simulink model "Simulator_Unitree_A1"  (R2022b)
settings: Solver=VariableStepAuto  StartTime=0.0  StopTime=70  RelTol=1e-3
undefined symbols (not defined in the file or in its folder): g, h, Kwalk, stepHeight, TsCtrl, tWalk, X, Y, Z
libraries: sm_lib x175, nesl_utility x69, simulink x2, slpidlib x2
(part 1 of 4)
settings Model: Creator=MUN  LastModifiedBy=MUN
settings ModelReferenceCC: EnableRefExpFcnMdlSchedulingChecks=on

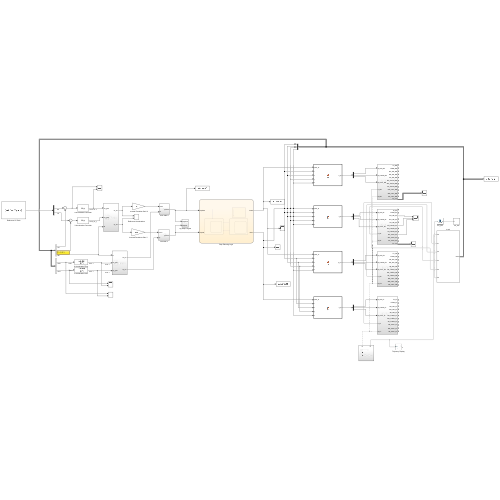
[thumbnail: Simulink's stored preview of the top-level diagram]
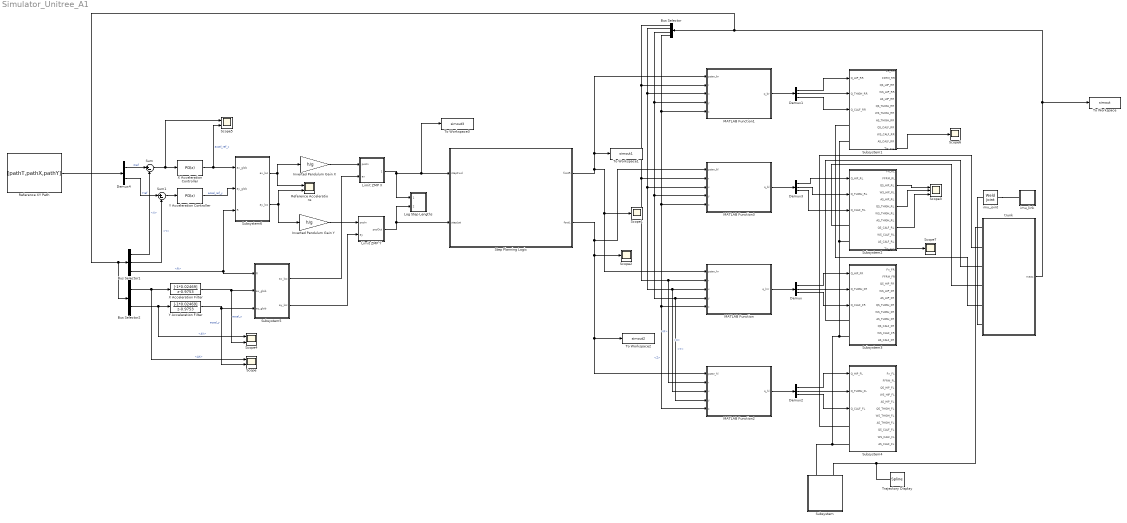
== system Simulator_Unitree_A1 ==
  Bus Selector : BusSelector  OutputSignals=R,X,Y,Z
  Bus Selector1 : BusSelector  OutputSignals=X,Y,R
  Bus Selector2 : BusSelector  OutputSignals=AX,AY
  Demux{,1..3} (4 alike) : Demux  Outputs=3
  Demux4 : Demux  Outputs=2
  Inverted Pendulum Gain X : Gain  Gain=h/g
  Inverted Pendulum Gain Y : Gain  Gain=h/g
  Limit ZMP X : Subsystem
  Limit ZMP Y : Subsystem
  Log Step Lengths : Subsystem
  MATLAB Function : MATLAB Function  TreatAsAtomicUnit=on
  MATLAB Function1 : MATLAB Function  TreatAsAtomicUnit=on
  MATLAB Function2 : MATLAB Function  TreatAsAtomicUnit=on
  MATLAB Function3 : MATLAB Function  TreatAsAtomicUnit=on
  Reference Accelerations : Scope  NumInputPorts=2
  Reference XY Path : FromWorkspace  VariableName=[pathT,pathX,pathY]  SampleTime=TsCtrl  OutputAfterFinalValue=Holding final value
  Scope : Scope  NumInputPorts=2
  Scope{1..2,6..7} (4 alike) : Scope
  Scope3 : Scope  NumInputPorts=3
  Scope4 : Scope  NumInputPorts=2
  Scope5 : Scope  NumInputPorts=2
  Step Planning Logic : Stateflow chart  TreatAsAtomicUnit=on
  Subsystem : Subsystem
  Subsystem1 : Subsystem
  Subsystem2 : Subsystem
  Subsystem3 : Subsystem
  Subsystem4 : Subsystem
  Subsystem5 : Subsystem
  Subsystem6 : Subsystem
  Sum : Sum  Inputs=|+-
  Sum1 : Sum  Inputs=|+-
  To Workspace : ToWorkspace  VariableName=simout  SaveFormat=Timeseries  SampleTime=-1
  To Workspace1 : ToWorkspace  VariableName=simout1  SaveFormat=Timeseries  SampleTime=-1
  To Workspace2 : ToWorkspace  VariableName=simout2  SaveFormat=Timeseries  SampleTime=-1
  To Workspace3 : ToWorkspace  VariableName=simout3  SaveFormat=Timeseries  SampleTime=-1
  Trajectory Display : sm_lib/Curves and Surfaces/Spline  GraphicAmbientColor=[0.15 0.15 0.15 1.0]  GraphicDiffuseColor=[0 0 0]  DataPoints=interPts  DataPointsUnits=m  GraphicEmissiveColor=[0.0 0.0 0.0 1.0]  EndConditionType=Natural  MarkerShape=Sphere  MarkerSize=10  GraphicType=FromGeometry  GraphicOpacity=1.0  GraphicShininess=75  GraphicSpecularColor=[0.5 0.5 0.5 1.0]  GraphicVisPropType=SimpleVisualProperties
  X Acceleration Controller : slpidlib/PID Controller  Controller=PD  Form=Parallel  TimeDomain=Discrete-time  UseExternalTs=off  SampleTime=-1  IntegratorMethod=Forward Euler  FilterMethod=Forward Euler  ControllerParametersSource=internal  P=3  I=0  UseKiTs=off  D=2  N=0.5  UseFilter=off  TunerSelectOption=Transfer Function Based (PID Tuner App)  InitialConditionSource=internal  InitialConditionForIntegrator=0  InitialConditionForFilter=0  DifferentiatorICPrevScaledInput=0  ExternalReset=none  TrackingMode=off  Kt=1  LimitOutput=off  SatLimitsSource=internal  UpperSaturationLimit=inf  LowerSaturationLimit=-inf  LinearizeAsGain=off  AntiWindupMode=none  Kb=1  LimitIntegrator=off  UpperIntegratorSaturationLimit=inf  LowerIntegratorSaturationLimit=-inf  POutMin=[]  POutMax=[]  IOutMin=[]  IOutMax=[]  DOutMin=[]  DOutMax=[]  NOutMin=[]  NOutMax=[]  SumOutMin=[]  SumOutMax=[]  SaturationOutMin=[]  SaturationOutMax=[]  PParamMin=[]  PParamMax=[]  IParamMin=[]  IParamMax=[]  DParamMin=[]  DParamMax=[]  NParamMin=[]  NParamMax=[]  KbParamMin=[]  KbParamMax=[]  KtParamMin=[]  KtParamMax=[]  KbOutMin=[]  KbOutMax=[]  KtOutMin=[]  KtOutMax=[]  IntegratorOutMin=[]  IntegratorOutMax=[]  FilterOutMin=[]  FilterOutMax=[]  SumI1OutMin=[]  SumI1OutMax=[]  SumI2OutMin=[]  SumI2OutMax=[]  SumI3OutMin=[]  SumI3OutMax=[]  SumI4OutMin=[]  SumI4OutMax=[]  SumDOutMin=[]  SumDOutMax=[]  DifferentiatorOutMin=[]  DifferentiatorOutMax=[]  FilterDiffOutCoefMin=[]  FilterDiffOutCoefMax=[]  ReciprocalOutMin=[]  ReciprocalOutMax=[]  SumDenOutMin=[]  SumDenOutMax=[]  SumNumOutMin=[]  SumNumOutMax=[]  DivideOutMin=[]  DivideOutMax=[]  UdiffTsProdOutMin=[]  UdiffTsProdOutMax=[]  NTsProdOutMin=[]  NTsProdOutMax=[]  UintegralTsProdOutMin=[]  UintegralTsProdOutMax=[]  UngainTsProdOutMin=[]  UngainTsProdOutMax=[]  ClampingZeroOutDataTypeStr=Inherit: Inherit via back propagation  ClampingZeroOutMin=[]  ClampingZeroOutMax=[]  FilterDenConstantOutDataTypeStr=Inherit: Inherit via back propagation  FilterDenConstantOutMin=[]  FilterDenConstantOutMax=[]  PCopyOutDataTypeStr=Inherit: Inherit via back propagation  PCopyOutMin=[]  PCopyOutMax=[]  NCopyOutDataTypeStr=Inherit: Inherit via back propagation  NCopyOutMin=[]  NCopyOutMax=[]  IntegratorContinuousStateAttributes=''  IntegratorStateMustResolveToSignalObject=off  IntegratorRTWStateStorageClass=Auto  FilterContinuousStateAttributes=''  FilterStateMustResolveToSignalObject=off  FilterRTWStateStorageClass=Auto  ParallelPVariant=InternalParameters  IdealPVariant=Disabled  IVariant=Disabled  DVariant=InternalParameters  IntegratorVariant=Disabled  SatVariant=Disabled  AWVariant=Disabled  PCopyVariant=Disabled  TRVariant=Disabled  FdbkBlocksVariant=Forward  IdealPFdbkVariant=Disabled  SatFdbkVariant=Disabled  DerivativeFilterVariant=Differentiator  NVariant=Passthrough  NCopyVariant=Disabled_SignalSpec  FilterICVariant=InternalICsDifferentiator  IntegratorICVariant=Disabled  ExternalResetVariant=Disabled  TRSumVariant=Passthrough  SumFdbkVariant=Disabled  SumVariant=Sum_PD  TsampFilterVariant=InternalTs  TsampNgainVariant=Passthrough  TsampIntegralVariant=Disabled_SignalSpec  ExternalSaturationOutDataTypeStr=Inherit: Same as second input
  X Acceleration Filter : DiscreteTransferFcn  Numerator=[-1*0.02469]  Denominator=[1 -0.9753]
  Y Acceleration Controller : slpidlib/PID Controller  Controller=PD  Form=Parallel  TimeDomain=Discrete-time  UseExternalTs=off  SampleTime=-1  IntegratorMethod=Forward Euler  FilterMethod=Forward Euler  ControllerParametersSource=internal  P=3  I=0  UseKiTs=off  D=2  N=0.5  UseFilter=off  TunerSelectOption=Transfer Function Based (PID Tuner App)  InitialConditionSource=internal  InitialConditionForIntegrator=0  InitialConditionForFilter=0  DifferentiatorICPrevScaledInput=0  ExternalReset=none  TrackingMode=off  Kt=1  LimitOutput=off  SatLimitsSource=internal  UpperSaturationLimit=inf  LowerSaturationLimit=-inf  LinearizeAsGain=off  AntiWindupMode=none  Kb=1  LimitIntegrator=off  UpperIntegratorSaturationLimit=inf  LowerIntegratorSaturationLimit=-inf  POutMin=[]  POutMax=[]  IOutMin=[]  IOutMax=[]  DOutMin=[]  DOutMax=[]  NOutMin=[]  NOutMax=[]  SumOutMin=[]  SumOutMax=[]  SaturationOutMin=[]  SaturationOutMax=[]  PParamMin=[]  PParamMax=[]  IParamMin=[]  IParamMax=[]  DParamMin=[]  DParamMax=[]  NParamMin=[]  NParamMax=[]  KbParamMin=[]  KbParamMax=[]  KtParamMin=[]  KtParamMax=[]  KbOutMin=[]  KbOutMax=[]  KtOutMin=[]  KtOutMax=[]  IntegratorOutMin=[]  IntegratorOutMax=[]  FilterOutMin=[]  FilterOutMax=[]  SumI1OutMin=[]  SumI1OutMax=[]  SumI2OutMin=[]  SumI2OutMax=[]  SumI3OutMin=[]  SumI3OutMax=[]  SumI4OutMin=[]  SumI4OutMax=[]  SumDOutMin=[]  SumDOutMax=[]  DifferentiatorOutMin=[]  DifferentiatorOutMax=[]  FilterDiffOutCoefMin=[]  FilterDiffOutCoefMax=[]  ReciprocalOutMin=[]  ReciprocalOutMax=[]  SumDenOutMin=[]  SumDenOutMax=[]  SumNumOutMin=[]  SumNumOutMax=[]  DivideOutMin=[]  DivideOutMax=[]  UdiffTsProdOutMin=[]  UdiffTsProdOutMax=[]  NTsProdOutMin=[]  NTsProdOutMax=[]  UintegralTsProdOutMin=[]  UintegralTsProdOutMax=[]  UngainTsProdOutMin=[]  UngainTsProdOutMax=[]  ClampingZeroOutDataTypeStr=Inherit: Inherit via back propagation  ClampingZeroOutMin=[]  ClampingZeroOutMax=[]  FilterDenConstantOutDataTypeStr=Inherit: Inherit via back propagation  FilterDenConstantOutMin=[]  FilterDenConstantOutMax=[]  PCopyOutDataTypeStr=Inherit: Inherit via back propagation  PCopyOutMin=[]  PCopyOutMax=[]  NCopyOutDataTypeStr=Inherit: Inherit via back propagation  NCopyOutMin=[]  NCopyOutMax=[]  IntegratorContinuousStateAttributes=''  IntegratorStateMustResolveToSignalObject=off  IntegratorRTWStateStorageClass=Auto  FilterContinuousStateAttributes=''  FilterStateMustResolveToSignalObject=off  FilterRTWStateStorageClass=Auto  ParallelPVariant=InternalParameters  IdealPVariant=Disabled  IVariant=Disabled  DVariant=InternalParameters  IntegratorVariant=Disabled  SatVariant=Disabled  AWVariant=Disabled  PCopyVariant=Disabled  TRVariant=Disabled  FdbkBlocksVariant=Forward  IdealPFdbkVariant=Disabled  SatFdbkVariant=Disabled  DerivativeFilterVariant=Differentiator  NVariant=Passthrough  NCopyVariant=Disabled_SignalSpec  FilterICVariant=InternalICsDifferentiator  IntegratorICVariant=Disabled  ExternalResetVariant=Disabled  TRSumVariant=Passthrough  SumFdbkVariant=Disabled  SumVariant=Sum_PD  TsampFilterVariant=InternalTs  TsampNgainVariant=Passthrough  TsampIntegralVariant=Disabled_SignalSpec  ExternalSaturationOutDataTypeStr=Inherit: Same as second input
  Y Acceleration Filter : DiscreteTransferFcn  Numerator=[-1*0.02469]  Denominator=[1 -0.9753]
  imu_joint : sm_lib/Joints/Weld Joint  JointMode=Normal  SenseConstraintForce=off  SenseConstraintForceX=off  SenseConstraintForceY=off  SenseConstraintForceZ=off  SenseConstraintTorque=off  SenseConstraintTorqueX=off  SenseConstraintTorqueY=off  SenseConstraintTorqueZ=off  SenseTotalForce=off  SenseTotalForceX=off  SenseTotalForceY=off  SenseTotalForceZ=off  SenseTotalTorque=off  SenseTotalTorqueX=off  SenseTotalTorqueY=off  SenseTotalTorqueZ=off  CompositeWrenchDir=FollowerOnBase  CompositeWrenchFrame=BaseFrame
  imu_link : Subsystem
  trunk : Subsystem
      settings: PortSchema="{\"entries\":[{\"content\":{\"sides\":[{\"content\":{\"connectorIds\":[\"Out1\"]},\"type\":\"ConnectorPlacement.EquallySpacedRectSide\",\"uuid\":\"7376a86a-8770-43a1-89a9-4e7813322353\"},{\"content\":{\"connectorIds\":[\"RConn1\",\"RConn2\",\"RConn3\",\"RConn4\",\"RConn5\",\"RConn6\"],\"side\":\"RIGHT\"},\"type\":\"ConnectorPlacement.EquallySpacedRectSide\",\"uuid\":\"180eba54-5c89-4d6d-8e58-15143fb194fc\"},{\"content\":{\"connectorIds\":[],\"side\":\"TOP\"},\"type\":\"ConnectorPlacement.EquallySpacedRectSide\",\"uuid\":\"86808b5f-7587-4320-85a4-2335862b1c59\"}]},\"type\":\"ConnectorPlacement.EquallySpacedConnector\",\"uuid\":\"b1910719-1a28-43ea-8867-88a05065806a\"}],\"packageUris\":[\"http://schema.mathworks.com/mf0/Connector/R2020b\"],\"version\":\"1.0\"}"
  wires:
  Bus Selector/1 -> MATLAB Function1/2(r), MATLAB Function2/2(r), MATLAB Function/2(r), MATLAB Function3/2(r)  "<R>"
  Bus Selector/2 -> MATLAB Function1/3(x), MATLAB Function2/3(x), MATLAB Function/3(x), MATLAB Function3/3(x)  "<X>"
  Bus Selector/3 -> MATLAB Function1/4(y), MATLAB Function2/4(y), MATLAB Function/4(y), MATLAB Function3/4(y)  "<Y>"
  Bus Selector/4 -> MATLAB Function1/5(z), MATLAB Function2/5(z), MATLAB Function/5(z), MATLAB Function3/5(z)  "<Z>"
  MATLAB Function/1(q_hrr) -> Demux/1
  Demux/1 -> Subsystem3/1(Q_HIP_FR)
  Demux/2 -> Subsystem3/2(Q_THIGH_FR)
  Demux/3 -> Subsystem3/3(Q_CALF_FR)
  MATLAB Function1/1(q_br) -> Demux1/1
  Demux1/1 -> Subsystem1/1(Q_HIP_RR)
  Demux1/2 -> Subsystem1/2(Q_THIGH_RR)
  Demux1/3 -> Subsystem1/3(Q_CALF_RR)
  Demux2/2 -> Subsystem4/2(Q_THIGH_FL)
  MATLAB Function2/1(q_hl) -> Demux2/1
  Demux2/3 -> Subsystem4/3(Q_CALF_FL)
  Demux2/1 -> Subsystem4/1(Q_HIP_FL)
  MATLAB Function3/1(q_bl) -> Demux3/1
  Demux3/1 -> Subsystem2/1(Q_HIP_RL)
  Demux3/2 -> Subsystem2/2(Q_THIGH_RL)
  Demux3/3 -> Subsystem2/3(Q_CALF_RL)
  Limit ZMP Y/1(posOut) -> Log Step Lengths/2(stepLat), Step Planning Logic/2(stepLat)
  Limit ZMP X/1(posOut) -> Log Step Lengths/1(stepFwd), To Workspace3/1, Step Planning Logic/1(stepFwd)
  Subsystem5/1(ax_loc) -> Limit ZMP X/2(ax)
  Y Acceleration Controller/1 -> Subsystem6/2(ay_glob)  "accel_ref_y"
  Subsystem5/2(ay_loc) -> Limit ZMP Y/2(ay)
  Inverted Pendulum Gain X/1 -> Limit ZMP X/1(posIn)
  Sum1/1 -> Y Acceleration Controller/1
  trunk/1(meas) -> To Workspace/1, Bus Selector2/1, Bus Selector1/1, Bus Selector/1
  Bus Selector1/3 -> Subsystem5/1(R), Subsystem6/3(R)  "<R>"
  Subsystem6/2(ay_loc) -> Reference Accelerations/2, Inverted Pendulum Gain Y/1
  Inverted Pendulum Gain Y/1 -> Limit ZMP Y/1(posIn)
  Subsystem6/1(ax_loc) -> Inverted Pendulum Gain X/1, Reference Accelerations/1
  Demux4/1 -> Sum/1  "Xref"
  Demux4/2 -> Sum1/1  "Yref"
  Reference XY Path/1 -> Demux4/1
  Bus Selector1/1 -> Sum/2  "<X>"
  Bus Selector1/2 -> Sum1/2  "<Y>"
  X Acceleration Controller/1 -> Scope5/2, Subsystem6/1(ax_glob)  "accel_ref_x"
  Step Planning Logic/2(footL) -> MATLAB Function3/1(pstar_bl), Scope2/1, MATLAB Function2/1(pstar_hl), To Workspace2/1
  Step Planning Logic/1(footR) -> MATLAB Function1/1(pstar_br), To Workspace1/1, MATLAB Function/1(pstar_hr), Scope1/1
  Subsystem2/3(QS_HIP_RL) -> Scope3/1
  Subsystem2/6(QS_THIGH_RL) -> Scope3/2
  Subsystem2/9(QS_CALF_RL) -> Scope3/3
  Bus Selector2/2 -> Scope4/1, Y Acceleration Filter/1  "<AY>"
  X Acceleration Filter/1 -> Scope4/2, Subsystem5/2(ax_glob)  "accel_x"
  Bus Selector2/1 -> Scope/1, X Acceleration Filter/1  "<AX>"
  Y Acceleration Filter/1 -> Scope/2, Subsystem5/3(ay_glob)  "accel_y"
  Sum/1 -> Scope5/1, X Acceleration Controller/1
  Subsystem1/12(Tip_xyz) -> Scope6/1
  Subsystem2/12(Tip_xyz) -> Scope7/1
  connections:
  Subsystem4/LConn2 -- Subsystem1/LConn2 -- Subsystem2/LConn2 -- Subsystem3/LConn2 -- Subsystem/LConn1
  Subsystem2/LConn1 -- trunk/RConn3
  Subsystem/LConn2 -- Trajectory Display/LConn1 -- trunk/RConn6
  imu_joint/LConn1 -- trunk/RConn1
  Subsystem1/LConn1 -- trunk/RConn2
  imu_joint/RConn1 -- imu_link/LConn1
  Subsystem4/LConn1 -- trunk/RConn5
  Subsystem3/LConn1 -- trunk/RConn4

== system Simulator_Unitree_A1/Limit ZMP X ==
  posIn : Inport
  ax : Inport  Port=2
  Bias1 : Bias  Bias=0.1  SaturateOnIntegerOverflow=off
  Bias2 : Bias  Bias=-0.1  SaturateOnIntegerOverflow=off
  Inverted Pendulum Gain : Gain  Gain=h/g
  Saturation Dynamic : simulink/Discontinuities/Saturation Dynamic  OutMin=[]  OutMax=[]  OutDataTypeStr=Inherit: Same as second input  OutDataType=fixdt(1, 16)  OutScaling=2^-10  DoSatur=off
  posOut : Outport  VectorParamsAs1DForOutWhenUnconnected=off
  wires:
  posIn/1 -> Saturation Dynamic/2
  Bias2/1 -> Saturation Dynamic/3
  Bias1/1 -> Saturation Dynamic/1
  ax/1 -> Inverted Pendulum Gain/1
  Saturation Dynamic/1 -> posOut/1
  Inverted Pendulum Gain/1 -> Bias1/1, Bias2/1

== system Simulator_Unitree_A1/Limit ZMP Y ==
  posIn : Inport
  ay : Inport  Port=2
  Bias3 : Bias  Bias=0.03  SaturateOnIntegerOverflow=off
  Bias4 : Bias  Bias=-0.03  SaturateOnIntegerOverflow=off
  Inverted Pendulum Gain : Gain  Gain=h/g
  Saturation Dynamic1 : simulink/Discontinuities/Saturation Dynamic  OutMin=[]  OutMax=[]  OutDataTypeStr=Inherit: Same as second input  OutDataType=fixdt(1, 16)  OutScaling=2^-10  DoSatur=off
  posOut : Outport  VectorParamsAs1DForOutWhenUnconnected=off
  wires:
  Bias4/1 -> Saturation Dynamic1/3
  Bias3/1 -> Saturation Dynamic1/1
  Inverted Pendulum Gain/1 -> Bias4/1, Bias3/1
  ay/1 -> Inverted Pendulum Gain/1
  posIn/1 -> Saturation Dynamic1/2
  Saturation Dynamic1/1 -> posOut/1

== system Simulator_Unitree_A1/Log Step Lengths ==
  stepFwd : Inport
  stepLat : Inport  Port=2
  Gain : Gain  Gain=100
  Gain1 : Gain  Gain=100
  Rate Transition : RateTransition  OutPortSampleTime=tWalk
  Rate Transition1 : RateTransition  OutPortSampleTime=tWalk
  Step Lengths [cm] : Scope  NumInputPorts=2
  wires:
  Rate Transition/1 -> Gain/1
  Gain/1 -> Step Lengths [cm]/1  "stepFwd"
  Gain1/1 -> Step Lengths [cm]/2  "stepLat"
  stepFwd/1 -> Rate Transition/1
  Rate Transition1/1 -> Gain1/1
  stepLat/1 -> Rate Transition1/1

== system Simulator_Unitree_A1/Subsystem ==
  MechanismConfiguration : sm_lib/Utilities/Mechanism Configuration  UniformGravity=Constant  GravityVector=[0 0 -9.80665]  GravityUnits=m/s^2  LinearizationDelta=0.001  JointModeTransitionNonlinearIterations=2
  Solver Configuration : nesl_utility/Solver Configuration  PhysicalDomain=network_engine_domain  SubClassName=solver  LeftPortType=input  RightPortType=generic  Tones=[]  Harmonics=[]  SimulateNoise=off  Profile=off  UseLocalSampling=off  EnableSwitchedLinearOptims=on  FrequencyDomain=off  UseCCode=off  RelTol=0.001  AbsTol=0.001  MinStep=1e-09  ToWorkspace=off  RevertToSquareIcSolve=off  NumHomotopyIterations=100  PhasorMode=off  PhasorModeNumHarmonics=1  ConsistencySolver=NEWTON_FTOL  IndexReductionMethod=DerivativeReplacement  DoDC=off  ResidualTolerance=1e-09  ConsistencyTolSource=GLOBAL  ConsistencyAbsTol=0.001  ConsistencyRelTol=0.001  ConsistencyTolFactor=0.001  UseLocalSolver=off  LocalSolverChoice=NE_BACKWARD_EULER_ADVANCER  ResolveIndetEquations=on  FunctionEvalNumThread=1  LocalSolverSampleTime=0.001  DoFixedCost=off  MaxNonlinIter=3  MaxModeIter=2  ComputeImpulses=off  ImpulseIterations=2  LinearAlgebra=auto  LinearAlgebraNumThread=0  EquationFormulation=NE_TIME_EF  DelaysMemoryBudget=1024  AutomaticFiltering=on  FilteringTimeConstant=0.001  PartitionStorageMethod=AS_NEEDED  PartitionMemoryBudget=1024  PartitionMethod=ROBUST
  Transform Floor Frame : sm_lib/Frames and Transforms/Rigid Transform  TranslationMethod=StandardAxis  TranslationStandardOffset=-0.06  TranslationLengthUnit=m  TranslationStandardAxis=+Z  TranslationCartesianOffset=[0 0 0]  TranslationROffset=0  TranslationROffsetUnits=m  TranslationZOffset=0  TranslationZOffsetUnits=m  TranslationThetaOffset=0  TranslationThetaOffsetUnits=deg  RotationMethod=None  RotationAngleUnits=deg  RotationStandardAxis=+X  RotationAngle=-90  RotationArbitraryAxis=[0 0 1]  FollAlignAxisA=+X  BaseAlignAxisA=+Y  FollAlignAxisB=+Y  BaseAlignAxisB=+Z  RotationSequenceAxes=FollowerAxes  RotationSequence=XYX  RotationSequenceAngles=[0 0 0]  RotationSequenceAnglesUnits=deg  RotationMatrix=[1 0 0; 0 1 0; 0 0 1]  Quaternion=[1 0 0 0]
  World : sm_lib/Frames and Transforms/World Frame
  World Plane : sm_lib/Body Elements/Brick Solid  GraphicAmbientColor=[0.15 0.15 0.15 1.0]  BasedOnType=Density  BrickDimensions=[5 5 0.1]  BrickDimensionUnits=m  CenterOfMass=[0 0 0]  CenterOfMassUnits=m  GraphicDiffuseColor=[0.2 0.2 1.0]  Density=1000  DensityUnits=kg/(m^3)  DoExposeReferenceFrame=on  GraphicEmissiveColor=[0.0 0.0 0.0 1.0]  ExportEntireGeometry=on  SerializedFrames=<Frames/>  MarkerShape=Sphere  MarkerSize=10  GraphicType=FromGeometry  InertiaType=CalculateFromGeometry  Mass=1  MassUnits=kg  MomentsOfInertia=[1 1 1]  MomentsOfInertiaUnits=kg*m^2  GraphicOpacity=0.5  ProductsOfInertia=[0 0 0]  ProductsOfInertiaUnits=kg*m^2  GraphicShininess=75  GraphicSpecularColor=[0.5 0.5 0.5 1.0]  GraphicVisPropType=SimpleVisualProperties
  G : PMIOPort  Side=Left
  W : PMIOPort  Port=2  Side=Left
  connections:
  Transform Floor Frame/LConn1 -- Solver Configuration/RConn1 -- MechanismConfiguration/RConn1 -- World/RConn1 -- W/RConn1
  World Plane/RConn1 -- Transform Floor Frame/RConn1
  World Plane/LConn1 -- G/RConn1

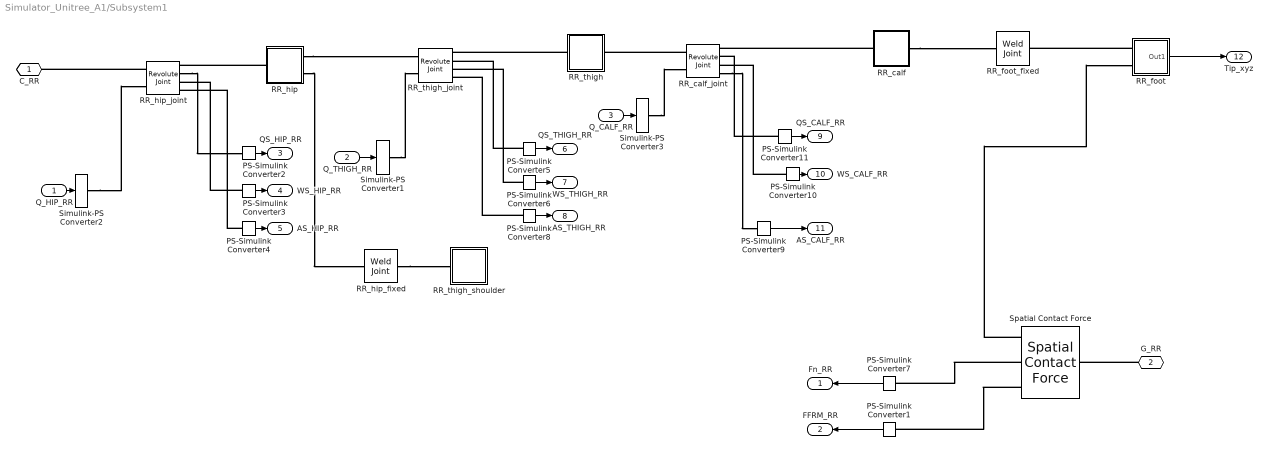
== system Simulator_Unitree_A1/Subsystem1 ==
  Q_HIP_RR : Inport
  Q_THIGH_RR : Inport  Port=2
  Q_CALF_RR : Inport  Port=3
  PS-Simulink Converter{1..11} (11 alike) : nesl_utility/PS-Simulink Converter  PhysicalDomain=network_engine_domain  SubClassName=ps_output  LeftPortType=input  RightPortType=output  PseudoPeriodic=off  Frequencies=[]  VectorFormat=1-D array  Unit=inherit  AffineConversion=off
  RR_calf : Subsystem
  RR_calf_joint : sm_lib/Joints/Revolute Joint  JointMode=Normal  SenseConstraintForce=off  SenseConstraintForceX=off  SenseConstraintForceY=off  SenseConstraintForceZ=off  SenseConstraintTorque=off  SenseConstraintTorqueX=off  SenseConstraintTorqueY=off  SenseConstraintTorqueZ=off  SenseTotalForce=off  SenseTotalForceX=off  SenseTotalForceY=off  SenseTotalForceZ=off  SenseTotalTorque=off  SenseTotalTorqueX=off  SenseTotalTorqueY=off  SenseTotalTorqueZ=off  CompositeWrenchDir=FollowerOnBase  CompositeWrenchFrame=BaseFrame  EquilibriumPosition=0  EquilibriumPositionUnits=deg  SpringStiffness=0  SpringStiffnessUnits=N*m/deg  DampingCoefficient=0.01  DampingCoefficientUnits=kg*m^2/(rad*s)  TorqueActuationMode=ComputedTorque  MotionActuationMode=InputMotion  SensePosition=on  SenseVelocity=on  SenseAcceleration=on  SenseTorqueForce=off  SenseLowerLimitTorqueForce=off  SenseUpperLimitTorqueForce=off  LowerLimitSpecify=on  LowerLimitBound=-2.69653369433  LowerLimitBoundUnits=rad  LowerLimitStiffness=1e4  LowerLimitStiffnessUnits=N*m/deg  LowerLimitDamping=10  LowerLimitDampingUnits=N*m/(deg/s)  LowerLimitTransitionRegionWidth=0.1  LowerLimitTransitionRegionWidthUnits=deg  UpperLimitSpecify=on  UpperLimitBound=-0.916297857297  UpperLimitBoundUnits=rad  UpperLimitStiffness=1e4  UpperLimitStiffnessUnits=N*m/deg  UpperLimitDamping=10  UpperLimitDampingUnits=N*m/(deg/s)  UpperLimitTransitionRegionWidth=0.1  UpperLimitTransitionRegionWidthUnits=deg  PositionTargetSpecify=on  PositionTargetPriority=High  PositionTargetValue=-1.7794  PositionTargetValueUnits=rad  VelocityTargetSpecify=off  VelocityTargetPriority=High  VelocityTargetValue=0  VelocityTargetValueUnits=deg/s
  RR_foot : Subsystem
  RR_foot_fixed : sm_lib/Joints/Weld Joint  JointMode=Normal  SenseConstraintForce=off  SenseConstraintForceX=off  SenseConstraintForceY=off  SenseConstraintForceZ=off  SenseConstraintTorque=off  SenseConstraintTorqueX=off  SenseConstraintTorqueY=off  SenseConstraintTorqueZ=off  SenseTotalForce=off  SenseTotalForceX=off  SenseTotalForceY=off  SenseTotalForceZ=off  SenseTotalTorque=off  SenseTotalTorqueX=off  SenseTotalTorqueY=off  SenseTotalTorqueZ=off  CompositeWrenchDir=FollowerOnBase  CompositeWrenchFrame=BaseFrame
  RR_hip : Subsystem
  RR_hip_fixed : sm_lib/Joints/Weld Joint  JointMode=Normal  SenseConstraintForce=off  SenseConstraintForceX=off  SenseConstraintForceY=off  SenseConstraintForceZ=off  SenseConstraintTorque=off  SenseConstraintTorqueX=off  SenseConstraintTorqueY=off  SenseConstraintTorqueZ=off  SenseTotalForce=off  SenseTotalForceX=off  SenseTotalForceY=off  SenseTotalForceZ=off  SenseTotalTorque=off  SenseTotalTorqueX=off  SenseTotalTorqueY=off  SenseTotalTorqueZ=off  CompositeWrenchDir=FollowerOnBase  CompositeWrenchFrame=BaseFrame
  RR_hip_joint : sm_lib/Joints/Revolute Joint  JointMode=Normal  SenseConstraintForce=off  SenseConstraintForceX=off  SenseConstraintForceY=off  SenseConstraintForceZ=off  SenseConstraintTorque=off  SenseConstraintTorqueX=off  SenseConstraintTorqueY=off  SenseConstraintTorqueZ=off  SenseTotalForce=off  SenseTotalForceX=off  SenseTotalForceY=off  SenseTotalForceZ=off  SenseTotalTorque=off  SenseTotalTorqueX=off  SenseTotalTorqueY=off  SenseTotalTorqueZ=off  CompositeWrenchDir=FollowerOnBase  CompositeWrenchFrame=BaseFrame  EquilibriumPosition=0  EquilibriumPositionUnits=deg  SpringStiffness=0  SpringStiffnessUnits=N*m/deg  DampingCoefficient=0.01  DampingCoefficientUnits=kg*m^2/(rad*s)  TorqueActuationMode=ComputedTorque  MotionActuationMode=InputMotion  SensePosition=on  SenseVelocity=on  SenseAcceleration=on  SenseTorqueForce=off  SenseLowerLimitTorqueForce=off  SenseUpperLimitTorqueForce=off  LowerLimitSpecify=on  LowerLimitBound=-0.802851455917  LowerLimitBoundUnits=rad  LowerLimitStiffness=1e4  LowerLimitStiffnessUnits=N*m/deg  LowerLimitDamping=10  LowerLimitDampingUnits=N*m/(deg/s)  LowerLimitTransitionRegionWidth=0.1  LowerLimitTransitionRegionWidthUnits=deg  UpperLimitSpecify=on  UpperLimitBound=0.802851455917  UpperLimitBoundUnits=rad  UpperLimitStiffness=1e4  UpperLimitStiffnessUnits=N*m/deg  UpperLimitDamping=10  UpperLimitDampingUnits=N*m/(deg/s)  UpperLimitTransitionRegionWidth=0.1  UpperLimitTransitionRegionWidthUnits=deg  PositionTargetSpecify=on  PositionTargetPriority=High  PositionTargetValue=0  PositionTargetValueUnits=rad  VelocityTargetSpecify=off  VelocityTargetPriority=High  VelocityTargetValue=0  VelocityTargetValueUnits=deg/s
  RR_thigh : Subsystem
  RR_thigh_joint : sm_lib/Joints/Revolute Joint  JointMode=Normal  SenseConstraintForce=off  SenseConstraintForceX=off  SenseConstraintForceY=off  SenseConstraintForceZ=off  SenseConstraintTorque=off  SenseConstraintTorqueX=off  SenseConstraintTorqueY=off  SenseConstraintTorqueZ=off  SenseTotalForce=off  SenseTotalForceX=off  SenseTotalForceY=off  SenseTotalForceZ=off  SenseTotalTorque=off  SenseTotalTorqueX=off  SenseTotalTorqueY=off  SenseTotalTorqueZ=off  CompositeWrenchDir=FollowerOnBase  CompositeWrenchFrame=BaseFrame  EquilibriumPosition=0  EquilibriumPositionUnits=deg  SpringStiffness=0  SpringStiffnessUnits=N*m/deg  DampingCoefficient=0.01  DampingCoefficientUnits=kg*m^2/(rad*s)  TorqueActuationMode=ComputedTorque  MotionActuationMode=InputMotion  SensePosition=on  SenseVelocity=on  SenseAcceleration=on  SenseTorqueForce=off  SenseLowerLimitTorqueForce=off  SenseUpperLimitTorqueForce=off  LowerLimitSpecify=on  LowerLimitBound=-1.0471975512  LowerLimitBoundUnits=rad  LowerLimitStiffness=1e4  LowerLimitStiffnessUnits=N*m/deg  LowerLimitDamping=10  LowerLimitDampingUnits=N*m/(deg/s)  LowerLimitTransitionRegionWidth=0.1  LowerLimitTransitionRegionWidthUnits=deg  UpperLimitSpecify=on  UpperLimitBound=4.18879020479  UpperLimitBoundUnits=rad  UpperLimitStiffness=1e4  UpperLimitStiffnessUnits=N*m/deg  UpperLimitDamping=10  UpperLimitDampingUnits=N*m/(deg/s)  UpperLimitTransitionRegionWidth=0.1  UpperLimitTransitionRegionWidthUnits=deg  PositionTargetSpecify=on  PositionTargetPriority=High  PositionTargetValue=0.7683  PositionTargetValueUnits=rad  VelocityTargetSpecify=off  VelocityTargetPriority=High  VelocityTargetValue=0  VelocityTargetValueUnits=deg/s
  RR_thigh_shoulder : Subsystem
  Simulink-PS Converter1 : nesl_utility/Simulink-PS Converter  PhysicalDomain=network_engine_domain  SubClassName=ps_input  LeftPortType=input  RightPortType=output  PseudoPeriodic=off  Frequencies=[]  NoiseDistribution=none  NoiseParameters=[]  Unit=1  AffineConversion=off  FilteringAndDerivatives=filter  SimscapeFilterOrder=2  InputFilterTimeConstant=tc  UdotUserProvided=0
  Simulink-PS Converter2 : nesl_utility/Simulink-PS Converter  PhysicalDomain=network_engine_domain  SubClassName=ps_input  LeftPortType=input  RightPortType=output  PseudoPeriodic=off  Frequencies=[]  NoiseDistribution=none  NoiseParameters=[]  Unit=1  AffineConversion=off  FilteringAndDerivatives=filter  SimscapeFilterOrder=2  InputFilterTimeConstant=tc  UdotUserProvided=0
  Simulink-PS Converter3 : nesl_utility/Simulink-PS Converter  PhysicalDomain=network_engine_domain  SubClassName=ps_input  LeftPortType=input  RightPortType=output  PseudoPeriodic=off  Frequencies=[]  NoiseDistribution=none  NoiseParameters=[]  Unit=1  AffineConversion=off  FilteringAndDerivatives=filter  SimscapeFilterOrder=2  InputFilterTimeConstant=tc  UdotUserProvided=0
  Spatial Contact Force : sm_lib/Forces and Torques/Spatial Contact Force  SenseContactBaseRotation=off  SenseContactBaseTranslation=off  CoefficientOfDynamicFriction=0.7  CoefficientOfStaticFriction=0.9  NormalDamping=damp  NormalDampingUnits=N/(m/s)  SenseContactSignal=off  NormalStiffness=stiff  NormalStiffnessUnits=N/m  FrictionalCriticalVelocity=0.01  FrictionalCriticalVelocityUnits=m/s  ZeroCrossDetectContactStartAndEnd=off  SenseContactFollowerRotation=off  SenseContactFollowerTranslation=off  FrictionType=SmoothStickSlip  SenseFrictionalForceMagnitude=on  SenseNormalForceMagnitude=on  NormalForceType=SmoothSpringDamper  SenseNormalVelocity=off  SenseSeparationDistance=off  SenseTangentialVelocity=off  NormalTransitionRegionWidth=1e-4  NormalTransitionRegionWidthUnits=m
  C_RR : PMIOPort  Side=Left
  G_RR : PMIOPort  Port=2  Side=Left
  Fn_RR : Outport
  FFRM_RR : Outport  Port=2
  QS_HIP_RR : Outport  Port=3
  WS_HIP_RR : Outport  Port=4
  AS_HIP_RR : Outport  Port=5
  QS_THIGH_RR : Outport  Port=6
  WS_THIGH_RR : Outport  Port=7
  AS_THIGH_RR : Outport  Port=8
  QS_CALF_RR : Outport  Port=9
  WS_CALF_RR : Outport  Port=10
  AS_CALF_RR : Outport  Port=11
  Tip_xyz : Outport  Port=12
  wires:
  PS-Simulink Converter7/1 -> Fn_RR/1
  PS-Simulink Converter1/1 -> FFRM_RR/1
  PS-Simulink Converter2/1 -> QS_HIP_RR/1
  PS-Simulink Converter3/1 -> WS_HIP_RR/1
  PS-Simulink Converter4/1 -> AS_HIP_RR/1
  PS-Simulink Converter5/1 -> QS_THIGH_RR/1
  PS-Simulink Converter6/1 -> WS_THIGH_RR/1
  PS-Simulink Converter8/1 -> AS_THIGH_RR/1
  PS-Simulink Converter9/1 -> AS_CALF_RR/1
  PS-Simulink Converter10/1 -> WS_CALF_RR/1
  PS-Simulink Converter11/1 -> QS_CALF_RR/1
  Q_CALF_RR/1 -> Simulink-PS Converter3/1
  Q_HIP_RR/1 -> Simulink-PS Converter2/1
  Q_THIGH_RR/1 -> Simulink-PS Converter1/1
  RR_foot/1(Out1) -> Tip_xyz/1
  connections:
  RR_calf/LConn1 -- RR_calf_joint/RConn1
  RR_hip/RConn2 -- RR_hip_fixed/LConn1
  PS-Simulink Converter5/LConn1 -- RR_thigh_joint/RConn2
  RR_calf/RConn1 -- RR_foot_fixed/LConn1
  RR_thigh/LConn1 -- RR_thigh_joint/RConn1
  RR_hip/RConn1 -- RR_thigh_joint/LConn1
  RR_hip_fixed/RConn1 -- RR_thigh_shoulder/LConn1
  RR_foot/LConn1 -- RR_foot_fixed/RConn1
  Simulink-PS Converter1/RConn1 -- RR_thigh_joint/LConn2
  Simulink-PS Converter2/RConn1 -- RR_hip_joint/LConn2
  RR_hip/LConn1 -- RR_hip_joint/RConn1
  RR_calf_joint/LConn1 -- RR_thigh/RConn1
  RR_hip_joint/LConn1 -- C_RR/RConn1
  PS-Simulink Converter4/LConn1 -- RR_hip_joint/RConn4
  RR_hip_joint/RConn2 -- PS-Simulink Converter2/LConn1
  PS-Simulink Converter3/LConn1 -- RR_hip_joint/RConn3
  PS-Simulink Converter6/LConn1 -- RR_thigh_joint/RConn3
  PS-Simulink Converter8/LConn1 -- RR_thigh_joint/RConn4
  Spatial Contact Force/RConn2 -- PS-Simulink Converter7/LConn1
  Spatial Contact Force/RConn3 -- PS-Simulink Converter1/LConn1
  G_RR/RConn1 -- Spatial Contact Force/LConn1
  Spatial Contact Force/RConn1 -- RR_foot/LConn2
  RR_calf_joint/RConn4 -- PS-Simulink Converter9/LConn1
  PS-Simulink Converter10/LConn1 -- RR_calf_joint/RConn3
  PS-Simulink Converter11/LConn1 -- RR_calf_joint/RConn2
  Simulink-PS Converter3/RConn1 -- RR_calf_joint/LConn2

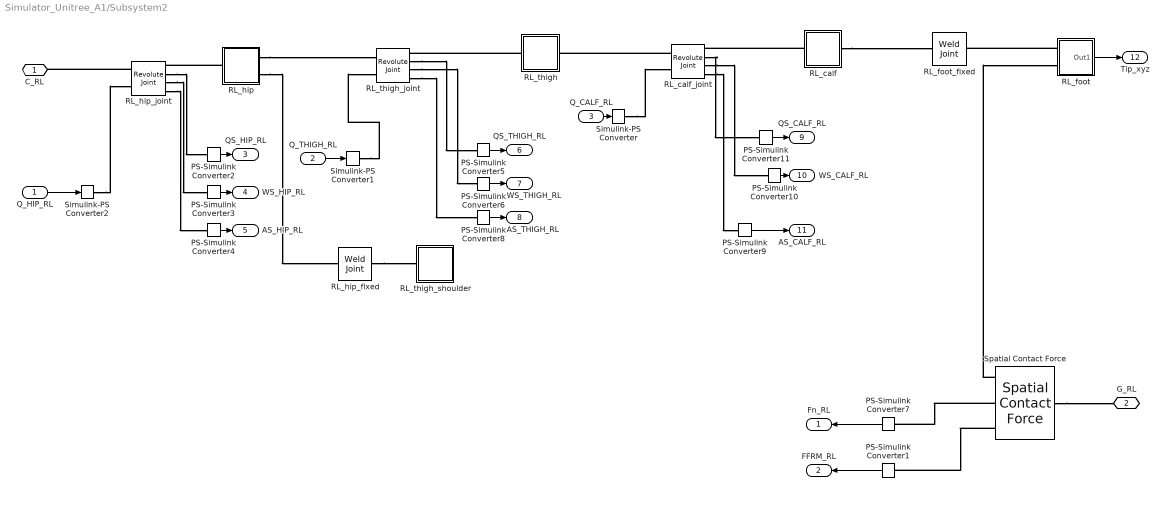
== system Simulator_Unitree_A1/Subsystem2 ==
  Q_HIP_RL : Inport
  Q_THIGH_RL : Inport  Port=2
  Q_CALF_RL : Inport  Port=3
  PS-Simulink Converter{1..11} (11 alike) : nesl_utility/PS-Simulink Converter  PhysicalDomain=network_engine_domain  SubClassName=ps_output  LeftPortType=input  RightPortType=output  PseudoPeriodic=off  Frequencies=[]  VectorFormat=1-D array  Unit=inherit  AffineConversion=off
  RL_calf : Subsystem
  RL_calf_joint : sm_lib/Joints/Revolute Joint  JointMode=Normal  SenseConstraintForce=off  SenseConstraintForceX=off  SenseConstraintForceY=off  SenseConstraintForceZ=off  SenseConstraintTorque=off  SenseConstraintTorqueX=off  SenseConstraintTorqueY=off  SenseConstraintTorqueZ=off  SenseTotalForce=off  SenseTotalForceX=off  SenseTotalForceY=off  SenseTotalForceZ=off  SenseTotalTorque=off  SenseTotalTorqueX=off  SenseTotalTorqueY=off  SenseTotalTorqueZ=off  CompositeWrenchDir=FollowerOnBase  CompositeWrenchFrame=BaseFrame  EquilibriumPosition=0  EquilibriumPositionUnits=deg  SpringStiffness=0  SpringStiffnessUnits=N*m/deg  DampingCoefficient=0.01  DampingCoefficientUnits=kg*m^2/(rad*s)  TorqueActuationMode=ComputedTorque  MotionActuationMode=InputMotion  SensePosition=on  SenseVelocity=on  SenseAcceleration=on  SenseTorqueForce=off  SenseLowerLimitTorqueForce=off  SenseUpperLimitTorqueForce=off  LowerLimitSpecify=on  LowerLimitBound=-2.69653369433  LowerLimitBoundUnits=rad  LowerLimitStiffness=1e4  LowerLimitStiffnessUnits=N*m/deg  LowerLimitDamping=10  LowerLimitDampingUnits=N*m/(deg/s)  LowerLimitTransitionRegionWidth=0.1  LowerLimitTransitionRegionWidthUnits=deg  UpperLimitSpecify=on  UpperLimitBound=-0.916297857297  UpperLimitBoundUnits=rad  UpperLimitStiffness=1e4  UpperLimitStiffnessUnits=N*m/deg  UpperLimitDamping=10  UpperLimitDampingUnits=N*m/(deg/s)  UpperLimitTransitionRegionWidth=0.1  UpperLimitTransitionRegionWidthUnits=deg  PositionTargetSpecify=on  PositionTargetPriority=High  PositionTargetValue=-1.7794  PositionTargetValueUnits=rad  VelocityTargetSpecify=off  VelocityTargetPriority=High  VelocityTargetValue=0  VelocityTargetValueUnits=deg/s
  RL_foot : Subsystem
  RL_foot_fixed : sm_lib/Joints/Weld Joint  JointMode=Normal  SenseConstraintForce=off  SenseConstraintForceX=off  SenseConstraintForceY=off  SenseConstraintForceZ=off  SenseConstraintTorque=off  SenseConstraintTorqueX=off  SenseConstraintTorqueY=off  SenseConstraintTorqueZ=off  SenseTotalForce=off  SenseTotalForceX=off  SenseTotalForceY=off  SenseTotalForceZ=off  SenseTotalTorque=off  SenseTotalTorqueX=off  SenseTotalTorqueY=off  SenseTotalTorqueZ=off  CompositeWrenchDir=FollowerOnBase  CompositeWrenchFrame=BaseFrame
  RL_hip : Subsystem
  RL_hip_fixed : sm_lib/Joints/Weld Joint  JointMode=Normal  SenseConstraintForce=off  SenseConstraintForceX=off  SenseConstraintForceY=off  SenseConstraintForceZ=off  SenseConstraintTorque=off  SenseConstraintTorqueX=off  SenseConstraintTorqueY=off  SenseConstraintTorqueZ=off  SenseTotalForce=off  SenseTotalForceX=off  SenseTotalForceY=off  SenseTotalForceZ=off  SenseTotalTorque=off  SenseTotalTorqueX=off  SenseTotalTorqueY=off  SenseTotalTorqueZ=off  CompositeWrenchDir=FollowerOnBase  CompositeWrenchFrame=BaseFrame
  RL_hip_joint : sm_lib/Joints/Revolute Joint  JointMode=Normal  SenseConstraintForce=off  SenseConstraintForceX=off  SenseConstraintForceY=off  SenseConstraintForceZ=off  SenseConstraintTorque=off  SenseConstraintTorqueX=off  SenseConstraintTorqueY=off  SenseConstraintTorqueZ=off  SenseTotalForce=off  SenseTotalForceX=off  SenseTotalForceY=off  SenseTotalForceZ=off  SenseTotalTorque=off  SenseTotalTorqueX=off  SenseTotalTorqueY=off  SenseTotalTorqueZ=off  CompositeWrenchDir=FollowerOnBase  CompositeWrenchFrame=BaseFrame  EquilibriumPosition=0  EquilibriumPositionUnits=deg  SpringStiffness=0  SpringStiffnessUnits=N*m/deg  DampingCoefficient=0.01  DampingCoefficientUnits=kg*m^2/(rad*s)  TorqueActuationMode=ComputedTorque  MotionActuationMode=InputMotion  SensePosition=on  SenseVelocity=on  SenseAcceleration=on  SenseTorqueForce=off  SenseLowerLimitTorqueForce=off  SenseUpperLimitTorqueForce=off  LowerLimitSpecify=on  LowerLimitBound=-0.802851455917  LowerLimitBoundUnits=rad  LowerLimitStiffness=1e4  LowerLimitStiffnessUnits=N*m/deg  LowerLimitDamping=10  LowerLimitDampingUnits=N*m/(deg/s)  LowerLimitTransitionRegionWidth=0.1  LowerLimitTransitionRegionWidthUnits=deg  UpperLimitSpecify=on  UpperLimitBound=0.802851455917  UpperLimitBoundUnits=rad  UpperLimitStiffness=1e4  UpperLimitStiffnessUnits=N*m/deg  UpperLimitDamping=10  UpperLimitDampingUnits=N*m/(deg/s)  UpperLimitTransitionRegionWidth=0.1  UpperLimitTransitionRegionWidthUnits=deg  PositionTargetSpecify=on  PositionTargetPriority=High  PositionTargetValue=0  PositionTargetValueUnits=rad  VelocityTargetSpecify=off  VelocityTargetPriority=High  VelocityTargetValue=0  VelocityTargetValueUnits=deg/s
  RL_thigh : Subsystem
  RL_thigh_joint : sm_lib/Joints/Revolute Joint  JointMode=Normal  SenseConstraintForce=off  SenseConstraintForceX=off  SenseConstraintForceY=off  SenseConstraintForceZ=off  SenseConstraintTorque=off  SenseConstraintTorqueX=off  SenseConstraintTorqueY=off  SenseConstraintTorqueZ=off  SenseTotalForce=off  SenseTotalForceX=off  SenseTotalForceY=off  SenseTotalForceZ=off  SenseTotalTorque=off  SenseTotalTorqueX=off  SenseTotalTorqueY=off  SenseTotalTorqueZ=off  CompositeWrenchDir=FollowerOnBase  CompositeWrenchFrame=BaseFrame  EquilibriumPosition=0  EquilibriumPositionUnits=deg  SpringStiffness=0  SpringStiffnessUnits=N*m/deg  DampingCoefficient=0.01  DampingCoefficientUnits=kg*m^2/(rad*s)  TorqueActuationMode=ComputedTorque  MotionActuationMode=InputMotion  SensePosition=on  SenseVelocity=on  SenseAcceleration=on  SenseTorqueForce=off  SenseLowerLimitTorqueForce=off  SenseUpperLimitTorqueForce=off  LowerLimitSpecify=on  LowerLimitBound=-1.0471975512  LowerLimitBoundUnits=rad  LowerLimitStiffness=1e4  LowerLimitStiffnessUnits=N*m/deg  LowerLimitDamping=10  LowerLimitDampingUnits=N*m/(deg/s)  LowerLimitTransitionRegionWidth=0.1  LowerLimitTransitionRegionWidthUnits=deg  UpperLimitSpecify=on  UpperLimitBound=4.18879020479  UpperLimitBoundUnits=rad  UpperLimitStiffness=1e4  UpperLimitStiffnessUnits=N*m/deg  UpperLimitDamping=10  UpperLimitDampingUnits=N*m/(deg/s)  UpperLimitTransitionRegionWidth=0.1  UpperLimitTransitionRegionWidthUnits=deg  PositionTargetSpecify=on  PositionTargetPriority=High  PositionTargetValue=0.7683  PositionTargetValueUnits=rad  VelocityTargetSpecify=off  VelocityTargetPriority=High  VelocityTargetValue=0  VelocityTargetValueUnits=deg/s
  RL_thigh_shoulder : Subsystem
  Simulink-PS Converter : nesl_utility/Simulink-PS Converter  PhysicalDomain=network_engine_domain  SubClassName=ps_input  LeftPortType=input  RightPortType=output  PseudoPeriodic=off  Frequencies=[]  NoiseDistribution=none  NoiseParameters=[]  Unit=rad  AffineConversion=on  FilteringAndDerivatives=filter  SimscapeFilterOrder=2  InputFilterTimeConstant=tc  UdotUserProvided=0
  Simulink-PS Converter1 : nesl_utility/Simulink-PS Converter  PhysicalDomain=network_engine_domain  SubClassName=ps_input  LeftPortType=input  RightPortType=output  PseudoPeriodic=off  Frequencies=[]  NoiseDistribution=none  NoiseParameters=[]  Unit=1  AffineConversion=off  FilteringAndDerivatives=filter  SimscapeFilterOrder=2  InputFilterTimeConstant=tc  UdotUserProvided=0
  Simulink-PS Converter2 : nesl_utility/Simulink-PS Converter  PhysicalDomain=network_engine_domain  SubClassName=ps_input  LeftPortType=input  RightPortType=output  PseudoPeriodic=off  Frequencies=[]  NoiseDistribution=none  NoiseParameters=[]  Unit=rad  AffineConversion=on  FilteringAndDerivatives=filter  SimscapeFilterOrder=2  InputFilterTimeConstant=tc  UdotUserProvided=0
  Spatial Contact Force : sm_lib/Forces and Torques/Spatial Contact Force  SenseContactBaseRotation=off  SenseContactBaseTranslation=off  CoefficientOfDynamicFriction=0.7  CoefficientOfStaticFriction=0.9  NormalDamping=damp  NormalDampingUnits=N/(m/s)  SenseContactSignal=off  NormalStiffness=stiff  NormalStiffnessUnits=N/m  FrictionalCriticalVelocity=0.01  FrictionalCriticalVelocityUnits=m/s  ZeroCrossDetectContactStartAndEnd=off  SenseContactFollowerRotation=off  SenseContactFollowerTranslation=off  FrictionType=SmoothStickSlip  SenseFrictionalForceMagnitude=on  SenseNormalForceMagnitude=on  NormalForceType=SmoothSpringDamper  SenseNormalVelocity=off  SenseSeparationDistance=off  SenseTangentialVelocity=off  NormalTransitionRegionWidth=1e-4  NormalTransitionRegionWidthUnits=m
  C_RL : PMIOPort  Side=Left
  G_RL : PMIOPort  Port=2  Side=Left
  Fn_RL : Outport
  FFRM_RL : Outport  Port=2
  QS_HIP_RL : Outport  Port=3
  WS_HIP_RL : Outport  Port=4
  AS_HIP_RL : Outport  Port=5
  QS_THIGH_RL : Outport  Port=6
  WS_THIGH_RL : Outport  Port=7
  AS_THIGH_RL : Outport  Port=8
  QS_CALF_RL : Outport  Port=9
  WS_CALF_RL : Outport  Port=10
  AS_CALF_RL : Outport  Port=11
  Tip_xyz : Outport  Port=12
  wires:
  PS-Simulink Converter7/1 -> Fn_RL/1
  PS-Simulink Converter1/1 -> FFRM_RL/1
  PS-Simulink Converter2/1 -> QS_HIP_RL/1
  Q_HIP_RL/1 -> Simulink-PS Converter2/1
  PS-Simulink Converter3/1 -> WS_HIP_RL/1
  PS-Simulink Converter4/1 -> AS_HIP_RL/1
  PS-Simulink Converter5/1 -> QS_THIGH_RL/1
  PS-Simulink Converter8/1 -> AS_THIGH_RL/1
  PS-Simulink Converter6/1 -> WS_THIGH_RL/1
  Q_THIGH_RL/1 -> Simulink-PS Converter1/1
  PS-Simulink Converter11/1 -> QS_CALF_RL/1
  PS-Simulink Converter10/1 -> WS_CALF_RL/1
  PS-Simulink Converter9/1 -> AS_CALF_RL/1
  Q_CALF_RL/1 -> Simulink-PS Converter/1
  RL_foot/1(Out1) -> Tip_xyz/1
  connections:
  RL_hip/RConn1 -- RL_thigh_joint/LConn1
  RL_calf/RConn1 -- RL_foot_fixed/LConn1
  RL_calf/LConn1 -- RL_calf_joint/RConn1
  RL_hip/LConn1 -- RL_hip_joint/RConn1
  RL_hip_fixed/RConn1 -- RL_thigh_shoulder/LConn1
  RL_calf_joint/LConn1 -- RL_thigh/RConn1
  RL_foot/LConn1 -- RL_foot_fixed/RConn1
  RL_hip/RConn2 -- RL_hip_fixed/LConn1
  RL_thigh/LConn1 -- RL_thigh_joint/RConn1
  RL_hip_joint/LConn1 -- C_RL/RConn1
  Spatial Contact Force/RConn2 -- PS-Simulink Converter7/LConn1
  Spatial Contact Force/RConn3 -- PS-Simulink Converter1/LConn1
  Spatial Contact Force/LConn1 -- G_RL/RConn1
  Spatial Contact Force/RConn1 -- RL_foot/LConn2
  RL_hip_joint/RConn2 -- PS-Simulink Converter2/LConn1
  RL_hip_joint/RConn3 -- PS-Simulink Converter3/LConn1
  RL_hip_joint/RConn4 -- PS-Simulink Converter4/LConn1
  Simulink-PS Converter1/RConn1 -- RL_thigh_joint/LConn2
  RL_thigh_joint/RConn3 -- PS-Simulink Converter6/LConn1
  RL_thigh_joint/RConn4 -- PS-Simulink Converter8/LConn1
  RL_thigh_joint/RConn2 -- PS-Simulink Converter5/LConn1
  Simulink-PS Converter2/RConn1 -- RL_hip_joint/LConn2
  RL_calf_joint/RConn2 -- PS-Simulink Converter11/LConn1
  RL_calf_joint/RConn3 -- PS-Simulink Converter10/LConn1
  RL_calf_joint/RConn4 -- PS-Simulink Converter9/LConn1
  Simulink-PS Converter/RConn1 -- RL_calf_joint/LConn2
